simulink model "simple_svpwm"  (Simulink 7.5)
settings: Solver=ode45  StartTime=0.0  StopTime=0.1  RelTol=1e-3
InitFcn:
  | clc;
  | 
  | f=50;           % Reference frequency
  | fs=4000;      % Switching frequency
  | m=1;           % Modulation index
  | 
  | Ts=10e-6;    % Sampling time of devices
StopFcn:
  | close all;
  | figure(1);
  | plot(a(:,1),a(:,2),'-b',b(:,1),b(:,2),'-r');
  | axis equal;
  | grid;
  | title('Space Vector Trajectory');
  | clear;
  | clc;
libraries: powerlib x15, powerlib_extras x3, simulink x1
Description:
  | This model simulates a simple space vector pulse width modulation technique
  | and plot space vector trajectory as well.
  | 
  | Syed Abdul Rahman Kashif
  | EED, UET, Lahore, Pakistan
settings Model: Creator=Abdul Rahman Kashif  LastModifiedBy=Abdul Rahman Kashif

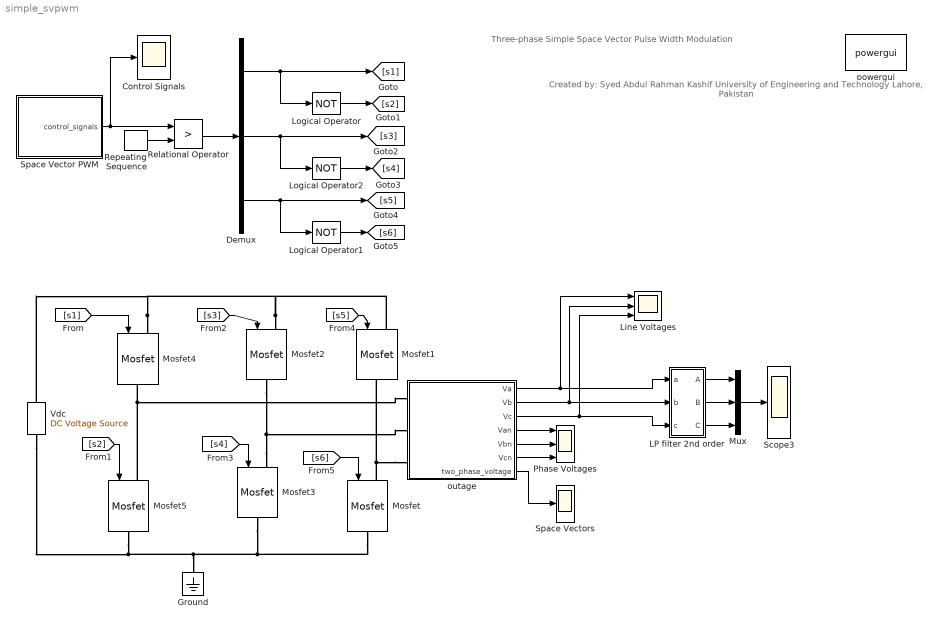
== system simple_svpwm ==
  note: Created by: Syed Abdul Rahman Kashif
      | University of Engineering and Technology
      | Lahore, Pakistan
  note: Three-phase Simple Space Vector Pulse Width Modulation
  Control Signals : Scope
      settings: TimeRange=0.02  YMin=-0.8  YMax=0.8  MaxDataPoints=25000  SampleInput=on  SampleTime=Ts
  Demux : Demux  Outputs=3
  Ground : powerlib/Elements/Ground  DialogController=POWERSYS.PowerSysDialog  PhysicalDomain=powersysdomain  SubClassName=unknown  LeftPortType=p1  RightPortType=p1  LConnTagsString=a
  LP filter 2nd order : Subsystem  mask{cutoff_frequency=200, damping_factor=0.707}
      mask prompts: cutoff_frequency "Cut off frequency"; damping_factor "Damping Factor"
  Line Voltages : Scope  NumInputPorts=3
      settings: YMin=-450~-450~-450  YMax=450~450~450  SaveName=Line_voltages  MaxDataPoints=5000000  SampleInput=on  SampleTime=2e-6
  Logical Operator : Logic  Operator=NOT  AllPortsSameDT=off  OutDataTypeMode=boolean  LogicDataType=fixdt(0, 8)  OutDataTypeStr=boolean
  Logical Operator1 : Logic  Operator=NOT  AllPortsSameDT=off  OutDataTypeMode=boolean  LogicDataType=fixdt(0, 8)  OutDataTypeStr=boolean
  Logical Operator2 : Logic  Operator=NOT  AllPortsSameDT=off  OutDataTypeMode=boolean  LogicDataType=fixdt(0, 8)  OutDataTypeStr=boolean
  Mosfet{,1..5} (6 alike) : powerlib/Power Electronics/Mosfet  DialogController=POWERSYS.PowerSysDialog  SystemSampleTime=-1  Ron=0.1  Lon=0  Rd=0.01  Vfd=0  IC=0  Rs=1e5  Cs=inf  Measurements=off
  Mux : Mux  Inputs=3
  Phase Voltages : Scope  NumInputPorts=3
      settings: YMin=-300~-300~-300  YMax=300~300~300  SaveName=Neutral_voltages  MaxDataPoints=5000000  SampleInput=on  SampleTime=2e-6
  Relational Operator : RelationalOperator  Operator=>
  Repeating Sequence : simulink/Sources/Repeating Sequence  SystemSampleTime=-1  rep_seq_t=[0 0.25/fs 0.5/fs 0.75/fs 1/fs]  rep_seq_y=[1 0 -1 0 1]
  Scope3 : Scope
      settings: YMin=-400  YMax=400  SaveName=Filtered_voltages  MaxDataPoints=5000000  SampleInput=on  SampleTime=2e-6
  Space Vector PWM : Subsystem
  Space Vectors : Scope
      settings: YMin=-350  YMax=350  SaveName=Neutral_voltages1  MaxDataPoints=5000000  SampleInput=on  SampleTime=2e-6
  Vdc : powerlib/Electrical Sources/DC Voltage Source  DialogController=POWERSYS.PowerSysDialog  SystemSampleTime=-1  Amplitude=400  Measurements=None
  outage : Subsystem
  powergui : powerlib/powergui  Priority=1  SystemSampleTime=-1  SimulationMode=Continuous  SampleTime=50e-6  frequency=60  SPID=off  DisableSnubberDevices=off  DisableRonSwitches=off  DisableVfSwitches=off  SwTol=0  Interpol=off  frequencyindice=0  echomessages=off  HookPort=off  DisplayEquations=off  FunctionMessages=off  EnableUseOfTLC=off  x0status=blocks  RestoreLinks=warning  ResistiveCurrentMeasurement=off  Ylog=off  Xlog=on  ShowGrid=off  save=off  variable=ZData  structure=Filtered_voltages  ZoomFFT=off  StartTime=0.02  cycles=1  DisplayStyle=1  fundamental=50  FreqAxis=off  MaxFrequency=1000  frequencyindicesteady=1  display=off  methode=off
  wires:
  Space Vector PWM/1(control_signals) -> Relational Operator/1, Control Signals/1
  Repeating Sequence/1 -> Relational Operator/2
  [s1] -> Mosfet4/1
  [s2] -> Mosfet5/1
  [s3] -> Mosfet2/1
  [s4] -> Mosfet3/1
  [s5] -> Mosfet1/1
  [s6] -> Mosfet/1
  outage/1(Va) -> LP filter 2nd order/1(a), Line Voltages/1
  outage/2(Vb) -> LP filter 2nd order/2(b), Line Voltages/2
  outage/3(Vc) -> LP filter 2nd order/3(c), Line Voltages/3
  outage/4(Van) -> Phase Voltages/1
  outage/5(Vbn) -> Phase Voltages/2
  outage/6(Vcn) -> Phase Voltages/3
  LP filter 2nd order/1(A) -> Mux/1
  LP filter 2nd order/2(B) -> Mux/2
  LP filter 2nd order/3(C) -> Mux/3
  Relational Operator/1 -> Demux/1
  Logical Operator/1 -> [s2]
  Logical Operator2/1 -> [s4]
  Logical Operator1/1 -> [s6]
  Demux/1 -> [s1], Logical Operator/1
  Demux/2 -> [s3], Logical Operator2/1
  Demux/3 -> [s5], Logical Operator1/1
  Mux/1 -> Scope3/1
  outage/7(two_phase_voltage) -> Space Vectors/1
  connections:
  Vdc/RConn1 -- Mosfet4/LConn1 -- Mosfet2/LConn1 -- Mosfet1/LConn1
  outage/LConn1 -- Mosfet4/RConn1 -- Mosfet5/LConn1
  outage/LConn3 -- Mosfet/LConn1 -- Mosfet1/RConn1
  Ground/LConn1 -- Mosfet/RConn1 -- Mosfet3/RConn1 -- Vdc/LConn1 -- Mosfet5/RConn1
  Mosfet3/LConn1 -- outage/LConn2 -- Mosfet2/RConn1

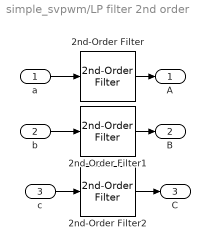
== system simple_svpwm/LP filter 2nd order ==
  a : Inport  OutDataType=sfix(16)  OutScaling=2^0
  b : Inport  Port=2  OutDataType=sfix(16)  OutScaling=2^0
  c : Inport  Port=3  OutDataType=sfix(16)  OutScaling=2^0
  2nd-Order Filter : powerlib_extras/Control  Blocks/2nd-Order Filter  DialogController=POWERSYS.PowerSysDialog  SystemSampleTime=-1  FilterType=Lowpass  Fo=cutoff_frequency  Zeta=damping_factor  Initialize=off  Vac_Init=[1 45 60]  Vdc_Init=-0.5  PlotResponse=off  param1=[1 500 1]
  2nd-Order Filter1 : powerlib_extras/Control  Blocks/2nd-Order Filter  DialogController=POWERSYS.PowerSysDialog  SystemSampleTime=-1  FilterType=Lowpass  Fo=cutoff_frequency  Zeta=damping_factor  Initialize=off  Vac_Init=[1 45 60]  Vdc_Init=-0.5  PlotResponse=off  param1=[1 500 1]
  2nd-Order Filter2 : powerlib_extras/Control  Blocks/2nd-Order Filter  DialogController=POWERSYS.PowerSysDialog  SystemSampleTime=-1  FilterType=Lowpass  Fo=cutoff_frequency  Zeta=damping_factor  Initialize=off  Vac_Init=[1 45 60]  Vdc_Init=-0.5  PlotResponse=off  param1=[1 500 1]
  A : Outport  OutDataType=sfix(16)  OutScaling=2^0
  B : Outport  Port=2  OutDataType=sfix(16)  OutScaling=2^0
  C : Outport  Port=3  OutDataType=sfix(16)  OutScaling=2^0
  wires:
  a/1 -> 2nd-Order Filter/1
  2nd-Order Filter/1 -> A/1
  b/1 -> 2nd-Order Filter1/1
  2nd-Order Filter1/1 -> B/1
  c/1 -> 2nd-Order Filter2/1
  2nd-Order Filter2/1 -> C/1

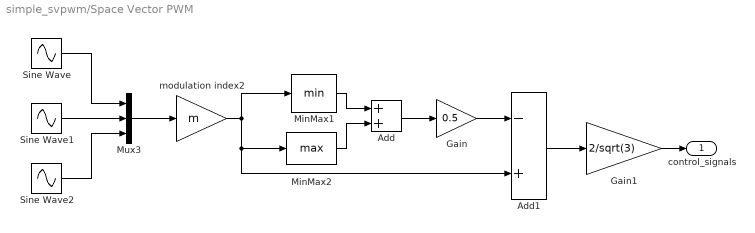
== system simple_svpwm/Space Vector PWM ==
  Add : Sum  OutDataType=fixdt(1, 16)  OutScaling=2^-10
  Add1 : Sum  Inputs=-+  OutDataType=fixdt(1, 16)  OutScaling=2^-10
  Gain : Gain  Gain=0.5  ParameterDataType=fixdt(1, 16)  ParameterScaling=2^0  OutDataType=fixdt(1, 16)  OutScaling=2^0
  Gain1 : Gain  Gain=2/sqrt(3)  ParameterDataType=fixdt(1, 16)  ParameterScaling=2^0  OutDataType=fixdt(1, 16)  OutScaling=2^0
  MinMax1 : MinMax  SaturateOnIntegerOverflow=on  InputSameDT=on
  MinMax2 : MinMax  Function=max  SaturateOnIntegerOverflow=on  InputSameDT=on
  Mux3 : Mux  Inputs=3
  Sine Wave : Sin  Amplitude=1  Bias=0  Frequency=2*pi*f  Phase=pi/2  Samples=10  SampleTime=0  Offset=0
  Sine Wave1 : Sin  Amplitude=1  Bias=0  Frequency=2*pi*f  Phase=pi/2 -2*pi/3  Samples=10  SampleTime=0  Offset=0
  Sine Wave2 : Sin  Amplitude=1  Bias=0  Frequency=2*pi*f  Phase=pi/2+2*pi/3  Samples=10  SampleTime=0  Offset=0
  modulation index2 : Gain  Gain=m  ParameterDataType=sfix(16)  ParameterScaling=2^0  OutDataType=sfix(16)  OutScaling=2^0  SaturateOnIntegerOverflow=on  OutDataTypeStr=Inherit: Same as input  ParamDataTypeStr=Inherit: Same as input
  control_signals : Outport
  wires:
  Sine Wave/1 -> Mux3/1
  Sine Wave1/1 -> Mux3/2
  Sine Wave2/1 -> Mux3/3
  Mux3/1 -> modulation index2/1
  modulation index2/1 -> MinMax1/1, MinMax2/1, Add1/2
  MinMax1/1 -> Add/1
  MinMax2/1 -> Add/2
  Add/1 -> Gain/1
  Gain/1 -> Add1/1
  Add1/1 -> Gain1/1
  Gain1/1 -> control_signals/1

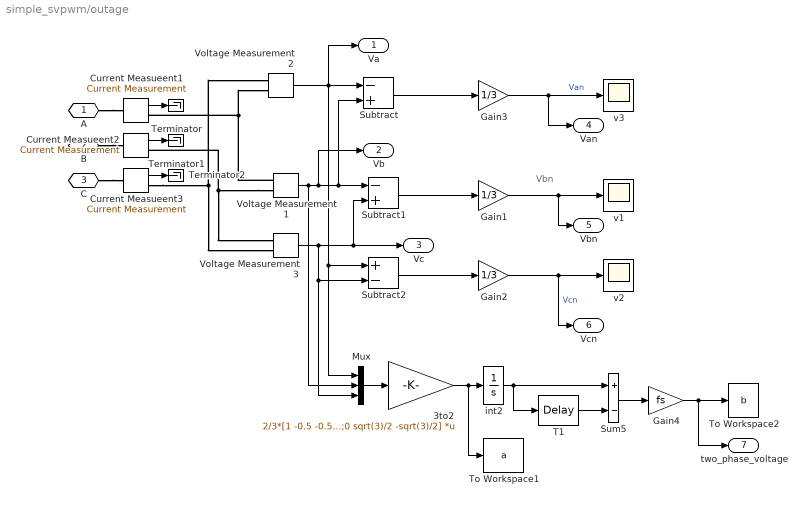
== system simple_svpwm/outage ==
  note: Vbn
  3to2 : Gain  Gain=2/3*[1 -0.5 -0.5;0 sqrt(3)/2 -sqrt(3)/2]  Multiplication=Matrix(K*u)  ParameterDataType=sfix(16)  ParameterScaling=2^0  OutDataType=sfix(16)  OutScaling=2^0  SaturateOnIntegerOverflow=on  OutDataTypeStr=Inherit: Same as input  ParamDataTypeStr=Inherit: Same as input
  Current Measueent1 : powerlib/Measurements/Current Measurement  DialogController=POWERSYS.PowerSysDialog  SystemSampleTime=-1  PhasorSimulation=off  OutputType=Complex  PSBequivalent=0
  Current Measueent2 : powerlib/Measurements/Current Measurement  DialogController=POWERSYS.PowerSysDialog  SystemSampleTime=-1  PhasorSimulation=off  OutputType=Complex  PSBequivalent=0
  Current Measueent3 : powerlib/Measurements/Current Measurement  DialogController=POWERSYS.PowerSysDialog  SystemSampleTime=-1  PhasorSimulation=off  OutputType=Complex  PSBequivalent=0
  Gain1 : Gain  Gain=1/3  ParameterDataType=sfix(16)  ParameterScaling=2^0  OutDataType=sfix(16)  OutScaling=2^0
  Gain2 : Gain  Gain=1/3  ParameterDataType=sfix(16)  ParameterScaling=2^0  OutDataType=sfix(16)  OutScaling=2^0
  Gain3 : Gain  Gain=1/3  ParameterDataType=sfix(16)  ParameterScaling=2^0  OutDataType=sfix(16)  OutScaling=2^0
  Gain4 : Gain  Gain=fs  ParameterDataType=sfix(16)  ParameterScaling=2^0  OutDataType=sfix(16)  OutScaling=2^0  SaturateOnIntegerOverflow=on  OutDataTypeStr=Inherit: Same as input  ParamDataTypeStr=Inherit: Same as input
  Mux : Mux  Inputs=3
  Subtract : Sum  Inputs=-+  OutDataType=sfix(16)  OutScaling=2^-10
  Subtract1 : Sum  Inputs=-+  OutDataType=sfix(16)  OutScaling=2^-10
  Subtract2 : Sum  Inputs=+-  OutDataType=sfix(16)  OutScaling=2^-10
  Sum5 : Sum  Inputs=+-  OutDataType=sfix(16)  OutScaling=2^0  SaturateOnIntegerOverflow=on  InputSameDT=on  OutDataTypeStr=Inherit: Same as first input
  T1 : TransportDelay  DelayTime=1/fs  BufferSize=2048
  Terminator : Terminator
  Terminator1 : Terminator
  Terminator2 : Terminator
  To Workspace1 : ToWorkspace  VariableName=a  SampleTime=-1  SaveFormat=Array
      settings: Decimation=2
  To Workspace2 : ToWorkspace  VariableName=b  SampleTime=-1  SaveFormat=Array
      settings: Decimation=2
  Voltage Measurement1 : powerlib/Measurements/Voltage Measurement  DialogController=POWERSYS.PowerSysDialog  SystemSampleTime=-1  PhasorSimulation=off  OutputType=Complex  PSBequivalent=0
  Voltage Measurement2 : powerlib/Measurements/Voltage Measurement  DialogController=POWERSYS.PowerSysDialog  SystemSampleTime=-1  PhasorSimulation=off  OutputType=Complex  PSBequivalent=0
  Voltage Measurement3 : powerlib/Measurements/Voltage Measurement  DialogController=POWERSYS.PowerSysDialog  SystemSampleTime=-1  PhasorSimulation=off  OutputType=Complex  PSBequivalent=0
  int2 : Integrator
  v1 : Scope
      settings: SaveName=ScopeData25  MaxDataPoints=5000000
  v2 : Scope
      settings: SaveName=ScopeData26  MaxDataPoints=5000000
  v3 : Scope
      settings: YMin=-300  YMax=300  SaveName=ScopeData27  MaxDataPoints=5000000
  A : PMIOPort  Port=1  Side=Left
  B : PMIOPort  Port=2  Side=Left
  C : PMIOPort  Port=3  Side=Left
  Va : Outport  OutDataType=sfix(16)  OutScaling=2^0
  Vb : Outport  Port=2  OutDataType=sfix(16)  OutScaling=2^0
  Vc : Outport  Port=3  OutDataType=sfix(16)  OutScaling=2^0
  Van : Outport  Port=4  OutDataType=sfix(16)  OutScaling=2^0
  Vbn : Outport  Port=5  OutDataType=sfix(16)  OutScaling=2^0
  Vcn : Outport  Port=6  OutDataType=sfix(16)  OutScaling=2^0
  two_phase_voltage : Outport  Port=7  OutDataType=sfix(16)  OutScaling=2^0
  wires:
  Gain2/1 -> v2/1, Vcn/1  "Vcn"
  Subtract2/1 -> Gain2/1
  Gain1/1 -> v1/1, Vbn/1
  Subtract1/1 -> Gain1/1
  Voltage Measurement3/1 -> Subtract1/2, Vc/1, Subtract2/2, Mux/3
  Gain3/1 -> v3/1, Van/1  "Van"
  Subtract/1 -> Gain3/1
  Voltage Measurement1/1 -> Subtract/2, Subtract1/1, Vb/1, Mux/2
  Voltage Measurement2/1 -> Subtract/1, Va/1, Subtract2/1, Mux/1
  Current Measueent1/1 -> Terminator/1
  Current Measueent2/1 -> Terminator1/1
  Current Measueent3/1 -> Terminator2/1
  Mux/1 -> 3to2/1
  3to2/1 -> int2/1, To Workspace1/1
  T1/1 -> Sum5/2
  int2/1 -> Sum5/1, T1/1
  Sum5/1 -> Gain4/1
  Gain4/1 -> To Workspace2/1, two_phase_voltage/1
  connections:
  Voltage Measurement1/LConn1 -- Current Measueent1/RConn1 -- Voltage Measurement2/LConn2
  Voltage Measurement1/LConn2 -- Current Measueent2/RConn1 -- Voltage Measurement3/LConn1
  Current Measueent3/RConn1 -- Voltage Measurement2/LConn1 -- Voltage Measurement3/LConn2
  A/RConn1 -- Current Measueent1/LConn1
  B/RConn1 -- Current Measueent2/LConn1
  C/RConn1 -- Current Measueent3/LConn1
